simulink model "process_and_retrieve"  (R2020a)
settings: Solver=FixedStepDiscrete  StartTime=0.0  StopTime=840000  RelTol=1e-3
libraries: hdlsllib x9, simulink x3
settings Model: FPTRunName=FPA_Reference  PacingRate=25  Creator=BuccelliLab  LastModifiedBy=diflo
settings SolverCC: AutoInsertRateTranBlk=on  MinimalZcImpactIntegration=on
settings DataIOCC: LimitDataPoints=on  SaveOutput=off  SaveTime=off  ReturnWorkspaceOutputs=off
settings OptimizationCC: BlockReduction=off  ConditionallyExecuteInputs=off  DefaultParameterBehavior=Inlined  LifeSpan=inf
settings DebuggingCC: SignalRangeChecking=warning  ReadBeforeWriteMsg=DisableAll  WriteAfterWriteMsg=DisableAll  WriteAfterReadMsg=DisableAll  AlgebraicLoopMsg=error  MultiTaskDSMMsg=none  SingleTaskRateTransMsg=error  ParameterDowncastMsg=warning  ParameterOverflowMsg=warning  AllowSymbolicDim=off  StrictBusMsg=ErrorOnBusTreatedAsVector  SFUnexpectedBacktrackingDiag=warning  SFNoUnconditionalDefaultTransitionDiag=warning  SFExecutionAtInitializationDiag=none  ArithmeticOperatorsInVariantConditions=warning
settings HardwareCC: ProdBitPerPointer=32  ProdBitPerSizeT=32  ProdBitPerPtrDiffT=32  ProdLargestAtomicFloat=None  ProdIntDivRoundTo=Undefined  ProdEndianess=Unspecified  ProdWordSize=32  ProdHWDeviceType=ASIC/FPGA->ASIC/FPGA  TargetBitPerPointer=64  TargetBitPerSizeT=64  TargetBitPerPtrDiffT=64  TargetLongLongMode=on  TargetIntDivRoundTo=Zero  TargetEndianess=LittleEndian  TargetWordSize=64  TargetHWDeviceType=Custom Processor->MATLAB Host Computer  ProdEqTarget=off
settings ModelReferenceCC: UpdateModelReferenceTargets=IfOutOfDate
settings SFSimCC: SFSimEcho=off  SimUseLocalCustomCode=off  CustomCodeUndefinedFunction=UseInterfaceOnly
settings RTWCC: RTWUseLocalCustomCode=off
settings CodeAppCC: StateflowObjectComments=on
settings GRTTargetCC: TargetLangStandard=C89/C90 (ANSI)
settings ConfigComp: CovScope=ReferencedModels  CovMetricSettings=dw  CovHtmlReporting=on  CovSaveCumulativeToWorkspaceVar=on  CovSaveSingleToWorkspaceVar=on  CovExternalEMLEnable=off  CovSFcnEnable=off

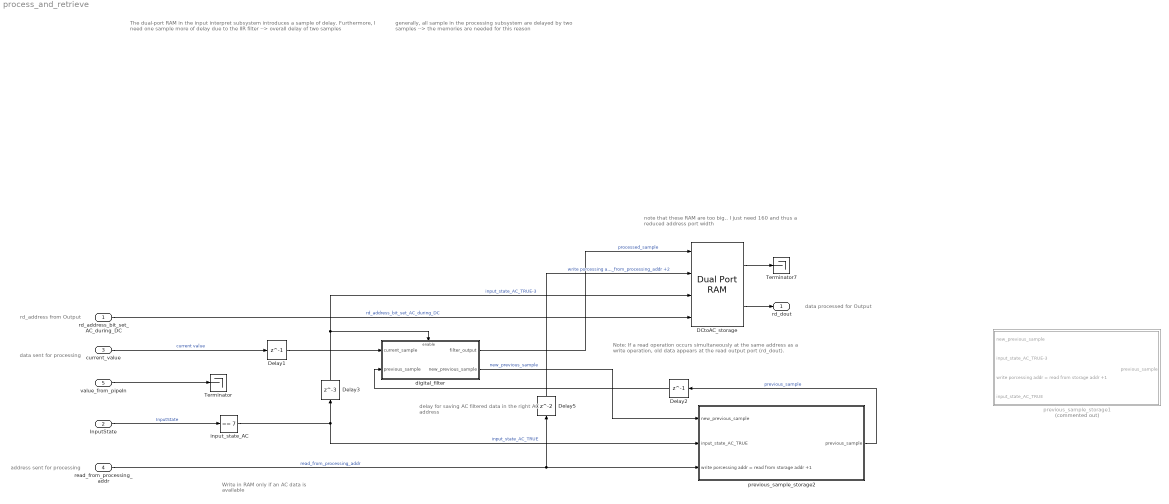
== system process_and_retrieve ==
  note: delay for saving AC filtered data in the right
      | AC address
  note: The dual-port RAM in the input interpret subsystem introduces
      | a sample of delay. Furthermore, I need one sample more of delay
      | due to the IIR filter --> overall delay of two samples
  note: generally, all sample in the processing subsystem
      | are delayed by two samples --> the memories are
      | needed for this reason
  note: data processed for Output
  note: rd_address from Output
  note: Write in RAM only if an AC data
      | is available
  note: note that these RAM are too big.. I just need 160 and thus a reduced address port width
  note: data sent for processing
  note: address sent for processing
  note: Note: If a read operation occurs simultaneously at the same address
      | as a write operation, old data appears at the read output port (rd_dout).
  rd_address_bit_set_AC_during_DC : Inport  OutDataTypeStr=fixdt(0,9,0)  PortDimensions=1  SampleTime=[1,0]
  InputState : Inport  Port=2  OutDataTypeStr=uint8  PortDimensions=1  SampleTime=[1,0]
  current_value : Inport  Port=3  OutDataTypeStr=uint16  PortDimensions=1  SampleTime=[1,0]
  read_from_processing_addr : Inport  Port=4  OutDataTypeStr=fixdt(0,9,0)  PortDimensions=1  SampleTime=[1,0]
  value_from_pipeIn : Inport  Port=5  OutDataTypeStr=uint16  PortDimensions=1  SampleTime=[1,0]
  DCtoAC_storage : hdlsllib/HDL RAMs/Dual Port RAM  ram_size=9
      settings: SourceProductBaseCode=SL
  Delay1 : Delay  DelayLength=1  InitialCondition=0
  Delay2 : Delay  DelayLength=1  InitialCondition=0
  Delay3 : Delay  DelayLength=3  InitialCondition=0
  Delay5 : Delay  InitialCondition=0
  Terminator : Terminator
  Terminator7 : Terminator
  digital_filter : Subsystem
  input_state_AC : simulink/Logic and Bit Operations/Compare To Constant  relop===  const=7  OutDataTypeStr=boolean
  previous_sample_storage1 : Subsystem  Commented=on
  previous_sample_storage2 : Subsystem
  rd_dout : Outport  OutDataTypeStr=uint16  PortDimensions=1  SampleTime=[1,0]
  wires:
  DCtoAC_storage/1 -> Terminator7/1
  rd_address_bit_set_AC_during_DC/1 -> DCtoAC_storage/4  "rd_address_bit_set_AC_during_DC"
  input_state_AC/1 -> Delay3/1, previous_sample_storage2/2(input_state_AC_TRUE)  "input_state_AC_TRUE"
  value_from_pipeIn/1 -> Terminator/1
  read_from_processing_addr/1 -> previous_sample_storage2/3(write porcessing addr = read from storage addr +1), Delay5/1  "read_from_processing_addr"
  DCtoAC_storage/2 -> rd_dout/1
  digital_filter/1(filter_output) -> DCtoAC_storage/1  "processed_sample"
  digital_filter/2(new_previous_sample) -> previous_sample_storage2/1(new_previous_sample)  "new_previous_sample"
  InputState/1 -> input_state_AC/1  "InputState"
  current_value/1 -> Delay1/1  "current value"
  Delay1/1 -> digital_filter/1(current_sample)
  previous_sample_storage2/1(previous_sample) -> Delay2/1  "previous_sample"
  Delay2/1 -> digital_filter/2(previous_sample)
  Delay5/1 -> DCtoAC_storage/2  "write porcessing addr = read_from_processing_addr +2"
  Delay3/1 -> DCtoAC_storage/3, digital_filter/Enable  "input_state_AC_TRUE-3"

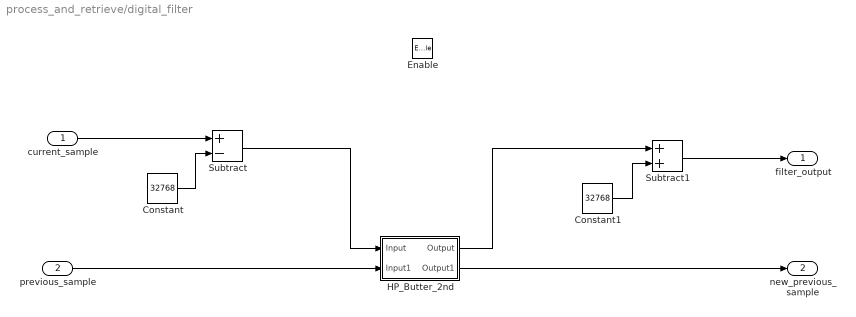
== system process_and_retrieve/digital_filter ==
  current_sample : Inport  OutDataTypeStr=fixdt(0,16,0)
  previous_sample : Inport  Port=2
  Enable : EnablePort
  Constant : Constant  Value=32768  OutDataTypeStr=fixdt(0,16,0)  SampleTime=-1
  Constant1 : Constant  Value=32768  OutDataTypeStr=fixdt(0,16,0)  SampleTime=-1
  HP_Butter_2nd : Subsystem  Tag=FilterWizardSubSystem
      settings: ErrorFcn=dspFilterRealizedInBasicElemsAlgLoopErrFcnCallback
  Subtract : Sum  Inputs=+-  OutDataTypeStr=fixdt(1,16,4)
  Subtract1 : Sum  OutDataTypeStr=fixdt(0,16,0)
  filter_output : Outport  InitialOutput=[0]
  new_previous_sample : Outport  Port=2  InitialOutput=[0]
  wires:
  HP_Butter_2nd/2(Output1) -> new_previous_sample/1
  previous_sample/1 -> HP_Butter_2nd/2(Input1)
  Subtract1/1 -> filter_output/1
  Constant1/1 -> Subtract1/2
  HP_Butter_2nd/1(Output) -> Subtract1/1
  current_sample/1 -> Subtract/1
  Subtract/1 -> HP_Butter_2nd/1(Input)
  Constant/1 -> Subtract/2

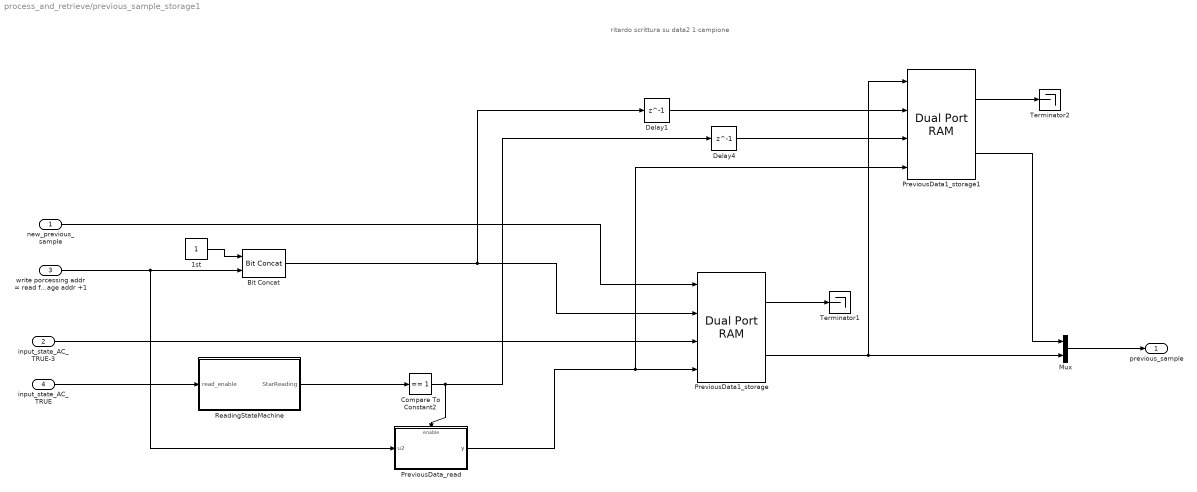
== system process_and_retrieve/previous_sample_storage1 ==
  note: ritardo scrittura su data2 1 campione
  new_previous_sample : Inport
  input_state_AC_TRUE-3 : Inport  Port=2
  write porcessing addr = read from storage addr +1 : Inport  Port=3
  input_state_AC_TRUE : Inport  Port=4
  1st : Constant  OutDataTypeStr=boolean  SampleTime=-1
  Bit Concat : hdlsllib/Logic and Bit Operations/Bit Concat  numInputs=2
  Compare To Constant2 : simulink/Logic and Bit Operations/Compare To Constant  relop===  const=1  OutDataTypeStr=boolean
  Delay1 : Delay  DelayLength=1  InitialCondition=0
  Delay4 : Delay  DelayLength=1  InitialCondition=0
  Mux : Mux  Inputs=2
  PreviousData1_storage : hdlsllib/HDL RAMs/Dual Port RAM  ram_size=10
      settings: SourceProductBaseCode=SL
  PreviousData1_storage1 : hdlsllib/HDL RAMs/Dual Port RAM  ram_size=10
      settings: SourceProductBaseCode=SL
  PreviousData_read : Subsystem
  ReadingStateMachine : Stateflow chart  TreatAsAtomicUnit=on
  Terminator1 : Terminator
  Terminator2 : Terminator
  previous_sample : Outport
  wires:
  Delay1/1 -> PreviousData1_storage1/2
  Delay4/1 -> PreviousData1_storage1/3
  PreviousData1_storage1/1 -> Terminator2/1
  Mux/1 -> previous_sample/1
  PreviousData1_storage1/2 -> Mux/1
  Compare To Constant2/1 -> Delay4/1, PreviousData_read/Enable
  ReadingStateMachine/1(StarReading) -> Compare To Constant2/1
  input_state_AC_TRUE/1 -> ReadingStateMachine/1(read_enable)
  PreviousData_read/1(y) -> PreviousData1_storage/4, PreviousData1_storage1/4
  write porcessing addr = read from storage addr +1/1 -> PreviousData_read/1(u2), Bit Concat/2
  input_state_AC_TRUE-3/1 -> PreviousData1_storage/3
  1st/1 -> Bit Concat/1
  PreviousData1_storage/2 -> Mux/2, PreviousData1_storage1/1
  new_previous_sample/1 -> PreviousData1_storage/1
  PreviousData1_storage/1 -> Terminator1/1
  Bit Concat/1 -> PreviousData1_storage/2, Delay1/1

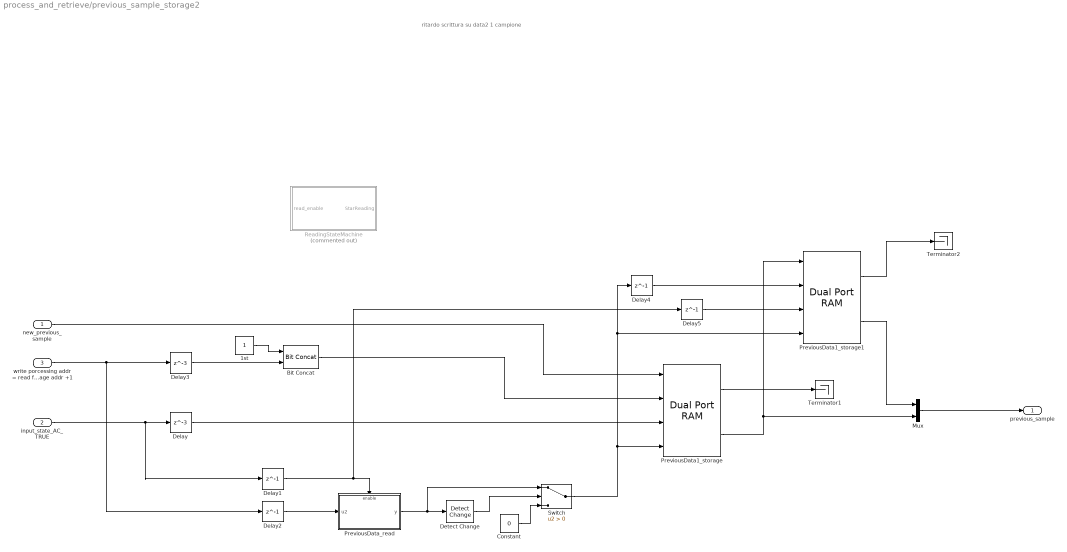
== system process_and_retrieve/previous_sample_storage2 ==
  note: ritardo scrittura su data2 1 campione
  new_previous_sample : Inport
  input_state_AC_TRUE : Inport  Port=2
  write porcessing addr = read from storage addr +1 : Inport  Port=3
  1st : Constant  OutDataTypeStr=boolean  SampleTime=-1
  Bit Concat : hdlsllib/Logic and Bit Operations/Bit Concat  numInputs=2
  Constant : Constant  Value=0  OutDataTypeStr=boolean  SampleTime=-1
  Delay : Delay  DelayLength=3  InitialCondition=0
  Delay{1..2,4..5} (4 alike) : Delay  DelayLength=1  InitialCondition=0
  Delay3 : Delay  DelayLength=3  InitialCondition=0
  Detect Change : simulink/Logic and Bit Operations/Detect Change  vinit=0  OutDataTypeStr=boolean
  Mux : Mux  Inputs=2
  PreviousData1_storage : hdlsllib/HDL RAMs/Dual Port RAM  ram_size=10
      settings: SourceProductBaseCode=SL
  PreviousData1_storage1 : hdlsllib/HDL RAMs/Dual Port RAM  ram_size=10
      settings: SourceProductBaseCode=SL
  PreviousData_read : Subsystem
  ReadingStateMachine : Stateflow chart  Commented=on  TreatAsAtomicUnit=on
  Switch : Switch  Criteria=u2 > Threshold
  Terminator1 : Terminator
  Terminator2 : Terminator
  previous_sample : Outport
  wires:
  Switch/1 -> PreviousData1_storage/4, PreviousData1_storage1/4, Delay4/1
  PreviousData_read/1(y) -> Detect Change/1, Switch/1
  Detect Change/1 -> Switch/2
  Constant/1 -> Switch/3
  Mux/1 -> previous_sample/1
  PreviousData1_storage1/2 -> Mux/1
  Delay5/1 -> PreviousData1_storage1/3
  PreviousData1_storage/2 -> PreviousData1_storage1/1, Mux/2
  PreviousData1_storage1/1 -> Terminator2/1
  Delay4/1 -> PreviousData1_storage1/2
  Delay3/1 -> Bit Concat/2
  Delay2/1 -> PreviousData_read/1(u2)
  Delay1/1 -> PreviousData_read/Enable, Delay5/1
  Delay/1 -> PreviousData1_storage/3
  write porcessing addr = read from storage addr +1/1 -> Delay3/1, Delay2/1
  input_state_AC_TRUE/1 -> Delay/1, Delay1/1
  1st/1 -> Bit Concat/1
  new_previous_sample/1 -> PreviousData1_storage/1
  PreviousData1_storage/1 -> Terminator1/1
  Bit Concat/1 -> PreviousData1_storage/2

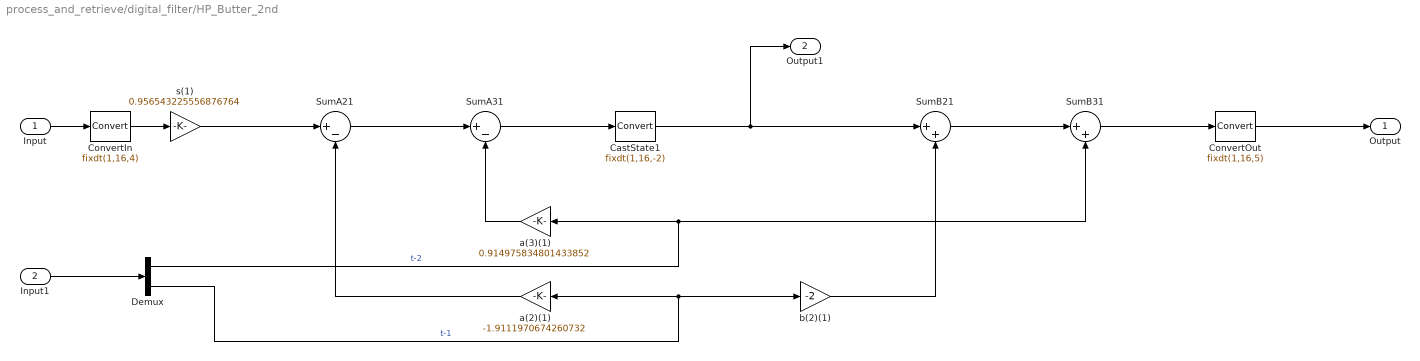
== system process_and_retrieve/digital_filter/HP_Butter_2nd ==
  Input : Inport  OutDataTypeStr=fixdt(1,16,4)
  Input1 : Inport  Port=2
  CastState1 : DataTypeConversion  OutDataTypeStr=fixdt(1,16,-2)  RndMeth=Convergent  SaturateOnIntegerOverflow=on
  ConvertIn : DataTypeConversion  OutDataTypeStr=fixdt(1,16,4)  RndMeth=Nearest  SaturateOnIntegerOverflow=on
  ConvertOut : DataTypeConversion  OutDataTypeStr=fixdt(1,16,5)  RndMeth=Convergent  SaturateOnIntegerOverflow=on
  Demux : Demux  Outputs=2
  SumA21 : Sum  Inputs=|+-  AccumDataTypeStr=fixdt(1,34,15)  OutDataTypeStr=fixdt(1,34,15)  RndMeth=Convergent  SaturateOnIntegerOverflow=on
  SumA31 : Sum  Inputs=|+-  AccumDataTypeStr=fixdt(1,34,15)  OutDataTypeStr=fixdt(1,34,16)  RndMeth=Convergent  SaturateOnIntegerOverflow=on
  SumB21 : Sum  Inputs=|++  AccumDataTypeStr=fixdt(1,34,15)  OutDataTypeStr=fixdt(1,34,16)  RndMeth=Convergent  SaturateOnIntegerOverflow=on
  SumB31 : Sum  Inputs=|++  AccumDataTypeStr=fixdt(1,34,16)  OutDataTypeStr=fixdt(1,34,23)  RndMeth=Convergent  SaturateOnIntegerOverflow=on
  a(2)(1) : Gain  Gain=-1.9111970674260732  ParamDataTypeStr=fixdt(1,16,14)  OutDataTypeStr=fixdt(1,32,13)  RndMeth=Convergent  SaturateOnIntegerOverflow=on
  a(3)(1) : Gain  Gain=0.914975834801433852  ParamDataTypeStr=fixdt(0,16,16)  OutDataTypeStr=fixdt(1,32,14)  RndMeth=Convergent  SaturateOnIntegerOverflow=on
  b(2)(1) : Gain  Gain=-2  ParamDataTypeStr=fixdt(1,16,14)  OutDataTypeStr=fixdt(1,32,13)  RndMeth=Convergent  SaturateOnIntegerOverflow=on
  s(1) : Gain  Gain=0.956543225556876764  ParamDataTypeStr=fixdt(0,16,16)  OutDataTypeStr=fixdt(1,16,4)  RndMeth=Convergent  SaturateOnIntegerOverflow=on
  Output : Outport
  Output1 : Outport  Port=2
  wires:
  Demux/2 -> a(2)(1)/1, b(2)(1)/1  "t-1"
  Demux/1 -> a(3)(1)/1, SumB31/2  "t-2"
  Input1/1 -> Demux/1
  ConvertIn/1 -> s(1)/1
  ConvertOut/1 -> Output/1
  a(3)(1)/1 -> SumA31/2
  b(2)(1)/1 -> SumB21/2
  a(2)(1)/1 -> SumA21/2
  SumB31/1 -> ConvertOut/1
  SumB21/1 -> SumB31/1
  CastState1/1 -> SumB21/1, Output1/1
  SumA31/1 -> CastState1/1
  SumA21/1 -> SumA31/1
  s(1)/1 -> SumA21/1
  Input/1 -> ConvertIn/1

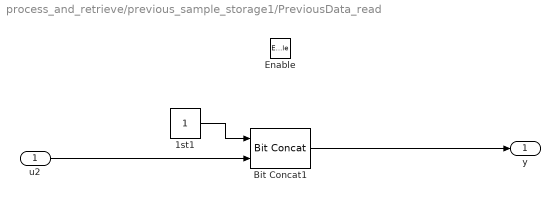
== system process_and_retrieve/previous_sample_storage1/PreviousData_read ==
  u2 : Inport
  Enable : EnablePort  StatesWhenEnabling=reset
  1st1 : Constant  OutDataTypeStr=boolean  SampleTime=-1
  Bit Concat1 : hdlsllib/Logic and Bit Operations/Bit Concat  numInputs=2
  y : Outport  OutputWhenDisabled=reset  InitialOutput=[0]
  wires:
  Bit Concat1/1 -> y/1
  1st1/1 -> Bit Concat1/1
  u2/1 -> Bit Concat1/2

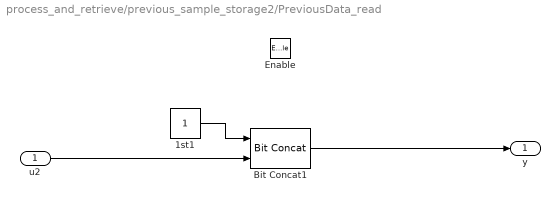
== system process_and_retrieve/previous_sample_storage2/PreviousData_read ==
  u2 : Inport
  Enable : EnablePort
  1st1 : Constant  OutDataTypeStr=boolean  SampleTime=-1
  Bit Concat1 : hdlsllib/Logic and Bit Operations/Bit Concat  numInputs=2
  y : Outport  InitialOutput=[0]
  wires:
  Bit Concat1/1 -> y/1
  1st1/1 -> Bit Concat1/1
  u2/1 -> Bit Concat1/2

== stateflow chart process_and_retrieve/previous_sample_storage1/ReadingStateMachine ==
  settings: sampleTime=1/1e6  stateMachineType=MOORE_MACHINE  initializeOutput=1
  state reading_idle1
    StarReading=0
  state reading_on
    StarReading=1
  (default) -> reading_idle1
  reading_on -> reading_idle1
  reading_idle1 -> reading_on : [read_enable == 1]
  data: StarReading output uint8; read_enable input

== stateflow chart process_and_retrieve/previous_sample_storage2/ReadingStateMachine ==
  settings: sampleTime=1/1e6  stateMachineType=MOORE_MACHINE  initializeOutput=1
  state reading_idle1
    StarReading=0
  state reading_on
    StarReading=1
  (default) -> reading_idle1
  reading_on -> reading_idle1
  reading_idle1 -> reading_on : [read_enable == 1]
  data: StarReading output uint8; read_enable input
